simulink model "onezonevav"  (R2020a)
settings: Solver=FixedStepAuto  StartTime=0.0  StopTime=Inf  FixedStep=0.001  RelTol=1e-3
PostLoadFcn:
  | if any(exist('dsrtsu_mdlpostloadfcn', 'file') ~= 0), dsrtsu_mdlpostloadfcn('Execute', bdroot); end
InitFcn:
  | , if any(exist('rtifpga_mdlclblib', 'file') ~= 0), rtifpga_mdlclblib('Init', bdroot); end,
  | , if any(exist('dsmpb_private', 'file') ~= 0), dsmpb_private('dsmpb_mdlclblib', 'Init', bdroot); end,
libraries: dsmpblib x4
(part 3 of 3)

== system onezonevav/behavior/dymola/Dymola Settings ==

== system onezonevav/behavior/dymola/Modelica model2 ==

== system onezonevav/behavior/dymola/compmodel ==

== system onezonevav/behavior/dymola/editmodel ==
